simulink model "SortPeriodSimulation"  (R2020b)
settings: Solver=VariableStepAuto  StartTime=0.0  StopTime=10.0  RelTol=1e-3
values from neighbouring files (symbols this model uses):
  actuatorDen = [1,   actuatorTimeConstant]    [generateAutopilotSmallPeriod.m]    (also in generateAutopilotVariables.m)
  actuatorNum = actuatorGain*actuatorTimeConstant    (= 5)    [generateAutopilotSmallPeriod.m]    (also in generateAutopilotVariables.m)
  AShortPeriod = AtotalLong(2:3,2:3)    [generateAutopilotSmallPeriod.m]    (also in generateAutopilotVariables.m = [-1.98701,   66.6537)
  BShortPeriod = [ -50.1873 ... (first row only)    [generateAutopilotSmallPeriod.m]    (also in generateAutopilotVariables.m = [-139.3498)
  CShortPeriod = [1,     0 ... (first row only)    [generateAutopilotSmallPeriod.m]    (also in generateAutopilotVariables.m)
  DShortPeriod = [0 ... (first row only)    [generateAutopilotSmallPeriod.m]    (also in generateAutopilotVariables.m)
  KDD = double(KDD)    [generateAutopilotVariables.m]
  KII = double(KII)    [generateAutopilotVariables.m]
  KPP = double(KPP)    [generateAutopilotVariables.m]
libraries: slpidlib x1
settings Model: Creator=Antonis Kantounias  LastModifiedBy=Antonis Kantounias

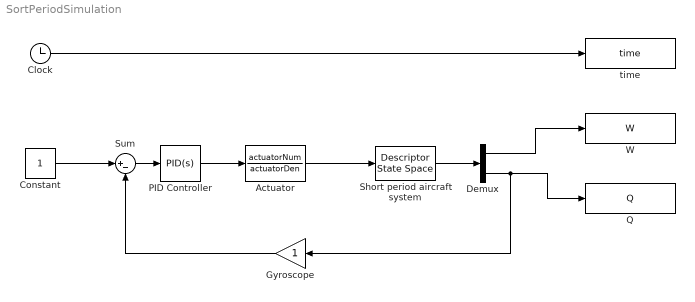
== system SortPeriodSimulation ==
  Actuator : TransferFcn  Numerator=actuatorNum  Denominator=actuatorDen
  Clock : Clock
  Constant : Constant
  Demux : Demux  Outputs=2
  Gyroscope : Gain
  PID Controller : slpidlib/PID Controller  Controller=PID  Form=Parallel  TimeDomain=Continuous-time  UseExternalTs=off  SampleTime=-1  IntegratorMethod=Forward Euler  FilterMethod=Forward Euler  ControllerParametersSource=internal  P=KPP  I=KII  D=KDD  UseFilter=on  N=100000  TunerSelectOption=Transfer Function Based (PID Tuner App)  InitialConditionSource=internal  InitialConditionForIntegrator=0  InitialConditionForFilter=0  DifferentiatorICPrevScaledInput=0  ExternalReset=none  TrackingMode=off  Kt=1  LimitOutput=off  SatLimitsSource=internal  UpperSaturationLimit=inf  LowerSaturationLimit=-inf  LinearizeAsGain=on  AntiWindupMode=none  Kb=1  POutMin=[]  POutMax=[]  IOutMin=[]  IOutMax=[]  DOutMin=[]  DOutMax=[]  NOutMin=[]  NOutMax=[]  SumOutMin=[]  SumOutMax=[]  SaturationOutMin=[]  SaturationOutMax=[]  PParamMin=[]  PParamMax=[]  IParamMin=[]  IParamMax=[]  DParamMin=[]  DParamMax=[]  NParamMin=[]  NParamMax=[]  KbParamMin=[]  KbParamMax=[]  KtParamMin=[]  KtParamMax=[]  KbOutMin=[]  KbOutMax=[]  KtOutMin=[]  KtOutMax=[]  IntegratorOutMin=[]  IntegratorOutMax=[]  FilterOutMin=[]  FilterOutMax=[]  SumI1OutMin=[]  SumI1OutMax=[]  SumI2OutMin=[]  SumI2OutMax=[]  SumI3OutMin=[]  SumI3OutMax=[]  SumI4OutMin=[]  SumI4OutMax=[]  SumDOutMin=[]  SumDOutMax=[]  DifferentiatorOutMin=[]  DifferentiatorOutMax=[]  FilterDiffOutCoefMin=[]  FilterDiffOutCoefMax=[]  ReciprocalOutMin=[]  ReciprocalOutMax=[]  SumDenOutMin=[]  SumDenOutMax=[]  SumNumOutMin=[]  SumNumOutMax=[]  DivideOutMin=[]  DivideOutMax=[]  UdiffTsProdOutMin=[]  UdiffTsProdOutMax=[]  NTsProdOutMin=[]  NTsProdOutMax=[]  UintegralTsProdOutMin=[]  UintegralTsProdOutMax=[]  UngainTsProdOutMin=[]  UngainTsProdOutMax=[]  IntegratorContinuousStateAttributes=''  IntegratorStateMustResolveToSignalObject=off  IntegratorRTWStateStorageClass=Auto  FilterContinuousStateAttributes=''  FilterStateMustResolveToSignalObject=off  FilterRTWStateStorageClass=Auto  ParallelPVariant=InternalParameters  IdealPVariant=Disabled  IVariant=InternalParameters  DVariant=InternalParameters  IntegratorVariant=Continuous  SatVariant=Disabled  AWVariant=Passthrough  PCopyVariant=Disabled  TRVariant=Disabled  FdbkBlocksVariant=Forward  IdealPFdbkVariant=Disabled  SatFdbkVariant=Disabled  DerivativeFilterVariant=ContFilter  NVariant=InternalParameters  NCopyVariant=Disabled  FilterICVariant=InternalICsFilter  IntegratorICVariant=InternalICs  ExternalResetVariant=Disabled  TRSumVariant=Passthrough  SumFdbkVariant=Disabled  SumVariant=Sum_PID  TsampFilterVariant=InternalTs  TsampNgainVariant=Passthrough  TsampIntegralVariant=Passthrough  ExternalSaturationOutDataTypeStr=Inherit: Same as second input
  Q : ToWorkspace  VariableName=Q  SaveFormat=Timeseries  SampleTime=-1
  Short period aircraft system : DescriptorStateSpace  E=EShordPeriod  A=AShortPeriod  B=BShortPeriod  C=CShortPeriod  D=DShortPeriod  InitialCondition=[0,0]
  Sum : Sum  Inputs=|+-
  W : ToWorkspace  VariableName=W  SaveFormat=Timeseries  SampleTime=-1
  time : ToWorkspace  VariableName=time  SaveFormat=Timeseries  SampleTime=-1
  wires:
  Clock/1 -> time/1
  Gyroscope/1 -> Sum/2
  Sum/1 -> PID Controller/1
  Demux/2 -> Gyroscope/1, Q/1
  Actuator/1 -> Short period aircraft system/1
  Constant/1 -> Sum/1
  PID Controller/1 -> Actuator/1
  Short period aircraft system/1 -> Demux/1
  Demux/1 -> W/1
